simulink model "accelerometer_test"  (R2022b)
settings: Solver=FixedStepAuto  StartTime=0.0  StopTime=inf  FixedStep=1e-3  RelTol=1e-3  EnableMultiTasking=on
undefined symbols (not defined in the file): magnitude
libraries: frdmk64flib x3, dspstat3 x3
settings Model: ExtModeTrigDuration=5  Creator=27161  LastModifiedBy=27161
settings SolverCC: AlgebraicLoopSolver=TrustRegion
settings OptimizationCC: EnhancedBackFolding=on  PassReuseOutputArgsAs=Individual arguments  ZeroExternalMemoryAtStartup=off  ZeroInternalMemoryAtStartup=off  MaxStackSize=64  OptimizeBlockOrder=speed  DifferentSizesBufferReuse=on  OptimizationCustomize=off  EfficientTunableParamExpr=on
settings DebuggingCC: ParameterTunabilityLossMsg=error  UnconnectedInputMsg=warning  UnconnectedOutputMsg=warning  UnconnectedLineMsg=warning  SFMachineParentedDataDiag=warning
settings HardwareCC: ProdBitPerPointer=32  ProdBitPerSizeT=32  ProdBitPerPtrDiffT=32  ProdLargestAtomicInteger=Long  ProdLargestAtomicFloat=Double  ProdWordSize=32  ProdHWDeviceType=ARM Compatible->ARM Cortex
settings ModelReferenceCC: EnableRefExpFcnMdlSchedulingChecks=on
settings SFSimCC: MATLABDynamicMemAlloc=off
settings RTWCC: Description=Embedded Coder  SystemTargetFile=ert.tlc  HardwareBoard=NXP FRDM-K64F  TLCOptions="-aInlineSetEventsForThisBaseRateFcn=TLC_FALSE -aSuppressMultiTaskScheduler=TLC_FALSE  -aRateBasedStepFcn=0"  TemplateMakefile=ert_default_tmf  Toolchain=GNU Tools for ARM Embedded Processors
settings CodeAppCC: ForceParamTrailComments=on  IgnoreCustomStorageClasses=off  OperatorAnnotations=on  SimulinkDataObjDesc=on  SFDataObjDesc=on  InsertBlockDesc=on

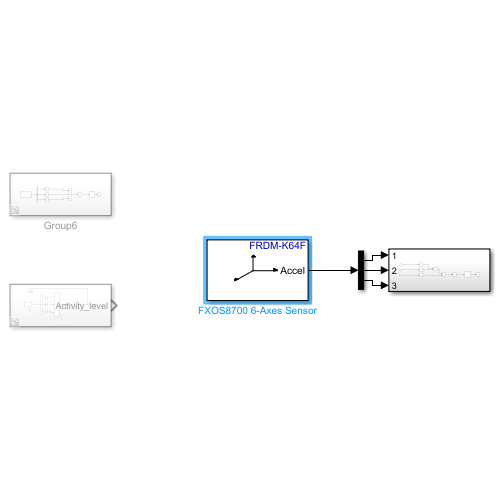
[thumbnail: Simulink's stored preview of the top-level diagram]
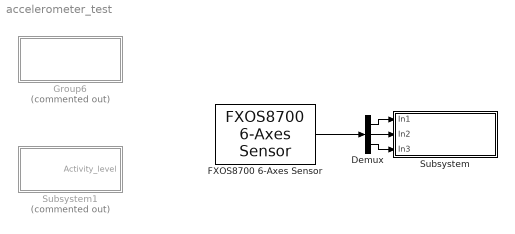
== system accelerometer_test ==
  Demux : Demux  Outputs=3
  FXOS8700 6-Axes Sensor : frdmk64flib/FXOS8700 6-Axes Sensor  Activesensor=Accelerometer only  ODR=800Hz  HybridODR=400Hz  Accelfullrange=-4g to +4g  SampleTime=0.1
  Group6 : Subsystem  Commented=on
  Subsystem : Subsystem
  Subsystem1 : Subsystem  Commented=on
  wires:
  Demux/1 -> Subsystem/1(In1)
  FXOS8700 6-Axes Sensor/1 -> Demux/1
  Demux/2 -> Subsystem/2(In2)
  Demux/3 -> Subsystem/3(In3)

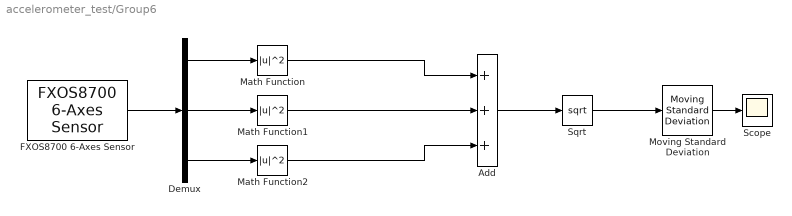
== system accelerometer_test/Group6 ==
  Add : Sum  Inputs=+++
  Demux : Demux  Outputs=3
  FXOS8700 6-Axes Sensor : frdmk64flib/FXOS8700 6-Axes Sensor  Activesensor=Accelerometer only  ODR=800Hz  HybridODR=400Hz  Accelfullrange=-4g to +4g  SampleTime=0.01
  Math Function : Math  Operator=magnitude^2  OutDataTypeStr=double
  Math Function1 : Math  Operator=magnitude^2  OutDataTypeStr=double
  Math Function2 : Math  Operator=magnitude^2  OutDataTypeStr=double
  Moving Standard Deviation : dspstat3/Moving Standard Deviation  Method=Sliding window  ForgettingFactorPort=off  SpecifyWindowLength=on  WindowLength=400  OverlapLength=399  AllowArbitraryInputLength=off  ForgettingFactor=0.9  SimulateUsing=Code generation
  Scope : Scope
  Sqrt : Sqrt  OutDataTypeStr=double  IntermediateResultsDataTypeStr=double
  wires:
  FXOS8700 6-Axes Sensor/1 -> Demux/1
  Moving Standard Deviation/1 -> Scope/1
  Sqrt/1 -> Moving Standard Deviation/1
  Demux/2 -> Math Function1/1
  Math Function/1 -> Add/1
  Demux/3 -> Math Function2/1
  Add/1 -> Sqrt/1
  Demux/1 -> Math Function/1
  Math Function1/1 -> Add/2
  Math Function2/1 -> Add/3

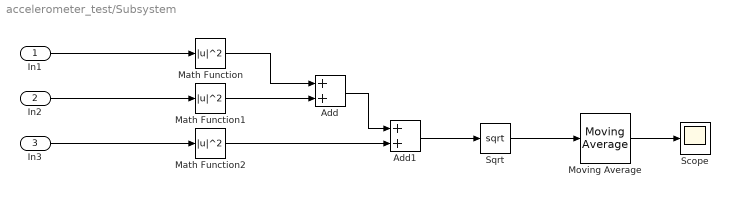
== system accelerometer_test/Subsystem ==
  In1 : Inport
  In2 : Inport  Port=2
  In3 : Inport  Port=3
  Add : Sum
  Add1 : Sum
  Math Function : Math  Operator=magnitude^2
  Math Function1 : Math  Operator=magnitude^2
  Math Function2 : Math  Operator=magnitude^2
  Moving Average : dspstat3/Moving Average  Method=Sliding window  ForgettingFactorPort=off  SpecifyWindowLength=on  WindowLength=600  OverlapLength=599  AllowArbitraryInputLength=off  ForgettingFactor=0.9  SimulateUsing=Code generation
  Scope : Scope
  Sqrt : Sqrt
  wires:
  In1/1 -> Math Function/1
  Math Function/1 -> Add/1
  In2/1 -> Math Function1/1
  Math Function1/1 -> Add/2
  In3/1 -> Math Function2/1
  Math Function2/1 -> Add1/2
  Add/1 -> Add1/1
  Add1/1 -> Sqrt/1
  Sqrt/1 -> Moving Average/1
  Moving Average/1 -> Scope/1

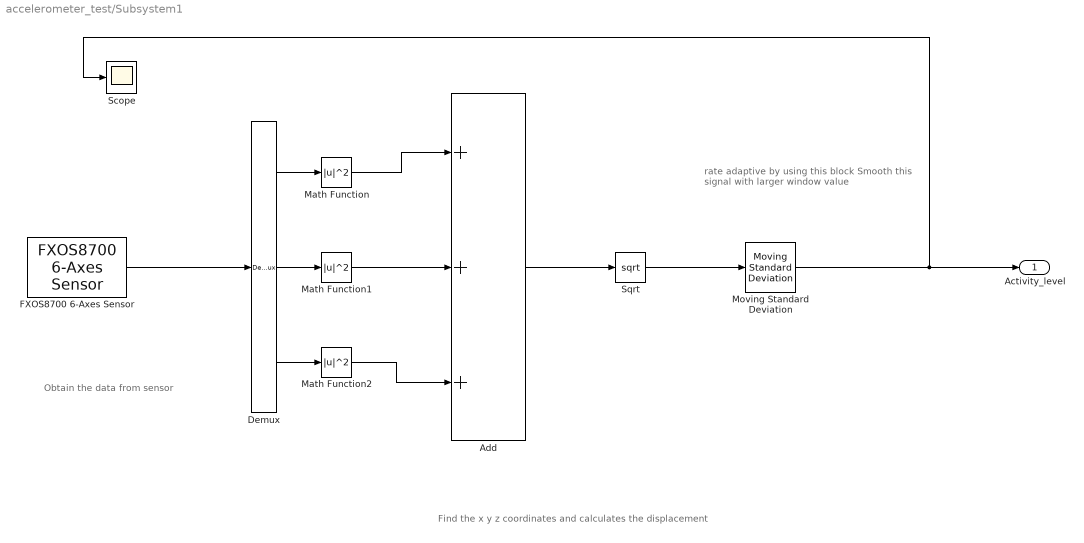
== system accelerometer_test/Subsystem1 ==
  note: Obtain the data from sensor
  note: Find the x y z coordinates and calculates the displacement
  note: rate adaptive by using this block
      | Smooth this signal with larger window value
  Add : Sum  Inputs=+++  OutDataTypeStr=double
  Demux : Demux  Outputs=3
  FXOS8700 6-Axes Sensor : frdmk64flib/FXOS8700 6-Axes Sensor  Activesensor=Accelerometer only  ODR=800Hz  HybridODR=400Hz  Accelfullrange=-4g to +4g  SampleTime=0.01
  Math Function : Math  Operator=magnitude^2  OutDataTypeStr=double
  Math Function1 : Math  Operator=magnitude^2  OutDataTypeStr=double
  Math Function2 : Math  Operator=magnitude^2  OutDataTypeStr=double
  Moving Standard Deviation : dspstat3/Moving Standard Deviation  Method=Sliding window  ForgettingFactorPort=off  SpecifyWindowLength=on  WindowLength=400  OverlapLength=399  AllowArbitraryInputLength=off  ForgettingFactor=0.9  SimulateUsing=Code generation
  Scope : Scope
  Sqrt : Sqrt  OutDataTypeStr=double
  Activity_level : Outport  OutDataTypeStr=double
  wires:
  Add/1 -> Sqrt/1
  Demux/2 -> Math Function1/1
  Math Function1/1 -> Add/2
  Sqrt/1 -> Moving Standard Deviation/1
  Demux/1 -> Math Function/1
  Math Function2/1 -> Add/3
  Math Function/1 -> Add/1
  Demux/3 -> Math Function2/1
  FXOS8700 6-Axes Sensor/1 -> Demux/1
  Moving Standard Deviation/1 -> Scope/1, Activity_level/1
